simulink library "AVE_Library"  (R2025b)
settings: Solver=VariableStepAuto  StartTime=0.0  StopTime=10.0  RelTol=1e-3
undefined symbols (not defined in the file or in its folder): DiscIntNeverNeededParam
libraries: simulink x44, etargetslib x18, $bdroot x13, GenericTarget x2
(part 2 of 5)

== system AVE_Library/Essential/Transformation ==
  Euler ZYX To Quaternion : Subsystem
      mask help: Convert Euler angles (ZYX-convention) to a unit quaternion. The order of the output quaternion is [W; XYZ], where W denotes the scalar part and XYZ denotes the vector part of the quaternion, respectively. The output quaternion indicates a rotation from b-frame to n-frame.
      mask DialogControl DescGroupVar Prompt: Euler (ZYX) To Quaternion
      mask Display: text(0.5, 0.5, 'Euler (ZYX)\nTo\nQuaternion', 'horizontalAlignment', 'center');
  Euler ZYX To Rotation Matrix : Subsystem
      mask help: Calculate the rotation matrix for a given roll, pitch and yaw angle (ZYX convention).
      mask DialogControl DescGroupVar Prompt: EulerZYXToRotationMatrix
      mask Display: disp('Euler (ZYX)\nTo\nRotation Matrix');
  LLA To NED : Subsystem
      mask help:
      | Convert LLA coordinates (WGS84) to local NED frame coordinates. This implementation uses the algorithm proposed by<br>
      | <i>S. P. Drake,
      | Converting GPS Coordinates to Navigation Coordinates,
      | Surveillance Systems Division, Electronics and Surveillance Research Laboratory, DSTO-TN-0432
      | April, 2002</i><br><br>
      |
      | <b>lat</b><br>Latitude (rad) of position that should be converted to NED.<br><br>
      | <b>lon</b><br>Longitude (rad) of position that should be converted to NED.<br><br>
      | <b>alt</b><br>Altitude (m, positive upwards) of position that should be converted to NED.<br><br>
      | <b>originLat</b><br>Latitude (rad) that indicates the origin of the local NED frame.<br><br>
      | <b>originLon</b><br>Longitude (rad) that indicates the origin of the local NED frame.<br><br>
      | <b>originAlt</b><br>Altitude (m, positive upwards) that indicates the origin of the local NED frame.
      mask DialogControl DescGroupVar Prompt: LLA To NED
      mask Display:
      | % Get dimension of block
      | pos = get_param(gcb, 'Position');
      | width = pos(3) - pos(1);
      | height = pos(4) - pos(2);
      | 
      | % Set image to center of block
      | image('AVE_Icon_LLA2NED.svg');
  LLA To NED Vector : Subsystem
      mask help:
      | Convert LLA coordinates (WGS84) to local NED frame coordinates. This implementation uses the algorithm proposed by<br>
      | <i>S. P. Drake,
      | Converting GPS Coordinates to Navigation Coordinates,
      | Surveillance Systems Division, Electronics and Surveillance Research Laboratory, DSTO-TN-0432
      | April, 2002</i><br><br>
      |
      | <b>positionLLA</b><br>Latitude (rad), longitude (rad) and altitude (m, positive upwards) of position that should be converted to NED.<br><br>
      | <b>originLLA</b><br>Latitude (rad), longitude (rad) and altitude (m, positive upwards) that indicates the origin of the local NED frame.
      mask DialogControl DescGroupVar Prompt: LLA To NED Vector
      mask Display:
      | % Get dimension of block
      | pos = get_param(gcb, 'Position');
      | width = pos(3) - pos(1);
      | height = pos(4) - pos(2);
      | 
      | % Set image to center of block
      | image('AVE_Icon_LLA2NEDVector.svg');
  NED To LLA : Subsystem
      mask help:
      | Convert local NED frame coordinates to LLA coordinates (WGS84). The altitude output is positive upwards.<br>
      | <br>
      | <b>N</b><br>North value of the NED position (m).<br><br>
      | <b>E</b><br>East value of the NED position (m).<br><br>
      | <b>D</b><br>Down value of the NED position (m).<br><br>
      | <b>originLat</b><br>Latitude (rad) that indicates the origin of the local NED frame.<br><br>
      | <b>originLon</b><br>Longitude (rad) that indicates the origin of the local NED frame.<br><br>
      | <b>originAlt</b><br>Altitude (m, positive upwards) that indicates the origin of the local NED frame.
      mask DialogControl DescGroupVar Prompt: NED To LLA
      mask Display:
      | % Get dimension of block
      | pos = get_param(gcb, 'Position');
      | width = pos(3) - pos(1);
      | height = pos(4) - pos(2);
      | 
      | % Set image to center of block
      | image('AVE_Icon_NED2LLA.svg');
  NED To LLA Vector : Subsystem
      mask help:
      | Convert local NED frame coordinates to LLA coordinates (WGS84). The altitude output is positive upwards.<br>
      | <br>
      | <b>positionNED</b><br>North, east and down value of the NED position (m).<br><br>
      | <b>originLLA</b><br>Latitude (rad), longitude (rad) and altitude (m, positive upwards) that indicates the origin of the local NED frame.
      mask DialogControl DescGroupVar Prompt: NED To LLA Vector
      mask Display:
      | % Get dimension of block
      | pos = get_param(gcb, 'Position');
      | width = pos(3) - pos(1);
      | height = pos(4) - pos(2);
      | 
      | % Set image to center of block
      | image('AVE_Icon_NED2LLAVector.svg');
  Quaternion To Euler ZYX : Subsystem
      mask help: Convert a unit quaternion to euler angles. The input quaternion indicates a rotation from b-frame to n-frame and is normalized by this function. The convention of rotation used is ZYX. The order of the input quaternion is [W; XYZ], where W denotes the scalar part and XYZ denotes the vector part of the quaternion, respectively.
      mask DialogControl DescGroupVar Prompt: Quaternion To Euler (ZYX)
      mask Display: text(0.5, 0.5, 'Quaternion\nTo\nEuler (ZYX)', 'horizontalAlignment', 'center');
  Quaternion To Rotation Matrix : Subsystem
      mask help: Convert a unit quaternion to a rotation matrix. The input quaternion indicates a rotation from b-frame to n-frame and is normalized by this function. The order of the input quaternion is [W; XYZ], where W denotes the scalar part and XYZ denotes the vector part of the quaternion, respectively. The output matrix indicates the rotation matrix from b-frame to n-frame.
      mask DialogControl DescGroupVar Prompt: Quaternion To Rotation Matrix
      mask Display: disp('Quaternion\nTo\nRotation Matrix');
  Transform Sensor Euler ZYX : Subsystem
      mask help:
      | Transform an orientation measurement given as euler angles (ZYX-convention) from the sensor-frame to the body frame.<br><br>
      | <b>rollSensor</b><br>Roll angle measurement of the sensor in rad w.r.t. the navigation frame, given in the sensor frame.<br><br>
      | <b>pitchSensor</b><br>Pitch angle measurement of the sensor in rad w.r.t. the navigation frame, given in the sensor frame.<br><br>
      | <b>yawSensor</b><br>Yaw angle measurement of the sensor in rad w.r.t. the navigation frame, given in the sensor frame.<br><br>
      | <b>R_b2s</b><br>Rotation matrix representing the rotation from body-frame to sensor-frame.<br><br>
      mask DialogControl DescGroupVar Prompt: Transform Sensor Velocity PQR
      mask Display: disp('Transform\nSensor\nEuler (ZYX)');
  Transform Sensor Position LLA : Subsystem
      mask help:
      | Transform a geographic position (WGS84) from sensor coordinates to a body-frame, e.g. GPS measurement to body origin.<br><br>
      | <b>latSensor</b><br>Latitude measurement of the sensor in radians.<br><br>
      | <b>lonSensor</b><br>Longitude measurement of the sensor in radians.<br><br>
      | <b>altSensor</b><br>Altitude measurement of the sensor in meters (positive upwards).<br><br>
      | <b>R_b2n</b><br>Rotation matrix representing the rotation from body-frame to navigation frame.<br><br>
      | <b>r_b2s</b><br>Vector that indicates the sensor position w.r.t. the body frame in body frame coordinates (meters).<br><br>
      mask DialogControl DescGroupVar Prompt: Transform Sensor Position LLA
      mask Display: disp('Transform\nSensor\nPosition');
  Transform Sensor Quaternion WXYZ : Subsystem
      mask help:
      | Transform a unit quaternion measurement from a sensor-frame to a body-frame.<br><br>
      | <table border="1" align="center" width="100%"><tr><th>Input</th></tr></table><br><br>
      | <b>quaternionSensor</b><br>
      | Input quaternion from sensor, representing orientation from sensor-frame with respect to navigation-frame.<br><br>
      |
      | <b>R_b2s</b><br>
      | 3-by-3 rotation matrix representing the rotation from body-frame to sensor-frame.<br><br>
      |
      | <table border="1" align="center" width="100%"><tr><th>Output</th></tr></table><br><br>
      | <b>quaternionBody</b><br>
      | Output unit quaternion in body-frame, representing the orientation from the body-frame with respect to the navigation frame.<br><br>
      mask DialogControl DescGroupVar Prompt: Transform Sensor Quaternion WXYZ
      mask Display: disp('Transform\nSensor\nQuaternion');
  Transform Sensor Velocity PQR : Subsystem
      mask help:
      | Transform an angular velocity measurement from a sensor-frame to a body-frame.<br><br>
      | <b>pSensor</b><br>P velocity measurement of the sensor in rad/s w.r.t. navigation frame.<br><br>
      | <b>qSensor</b><br>Q velocity measurement of the sensor in rad/s w.r.t. navigation frame.<br><br>
      | <b>rSensor</b><br>R velocity measurement of the sensor in rad/s w.r.t. navigation frame.<br><br>
      | <b>R_b2s</b><br>Rotation matrix representing the rotation from body-frame to sensor-frame.<br><br>
      mask DialogControl DescGroupVar Prompt: Transform Sensor Velocity PQR
      mask Display: disp('Transform\nSensor\nVelocity (PQR)');
  Transform Sensor Velocity UVW : Subsystem
      mask help:
      | Transform a velocity measurement from a sensor-frame to a body-frame, e.g. DVL measurement to body origin.<br><br>
      | <b>uSensor</b><br>U velocity measurement of the sensor in m/s w.r.t. navigation frame.<br><br>
      | <b>vSensor</b><br>V velocity measurement of the sensor in m/s w.r.t. navigation frame.<br><br>
      | <b>wSensor</b><br>W velocity measurement of the sensor in m/s w.r.t. navigation frame.<br><br>
      | <b>r_b2s</b><br>Vector that indicates the sensor position w.r.t. the body frame in body frame coordinates (meters).<br><br>
      | <b>R_b2s</b><br>Rotation matrix representing the rotation from body-frame to sensor-frame.<br><br>
      | <b>pqr</b><br>Vector of angular velocities in rad/s (angular rate of body-frame w.r.t. navigation-frame in b-frame coordinates).<br><br>
      mask DialogControl DescGroupVar Prompt: Transform Sensor Velocity UVW
      mask Display: disp('Transform\nSensor\nVelocity (UVW)');
  Yaw To Rotation Matrix : Subsystem
      mask help: Create 2-by-2 rotation matrix from given yaw angle. The output rotation matrix represents a transformation from body to navigation frame.
      mask DialogControl DescGroupVar Prompt: Yaw To Rotation Matrix
      mask Display: disp('Yaw\nTo\nRotation Matrix (2x2)');

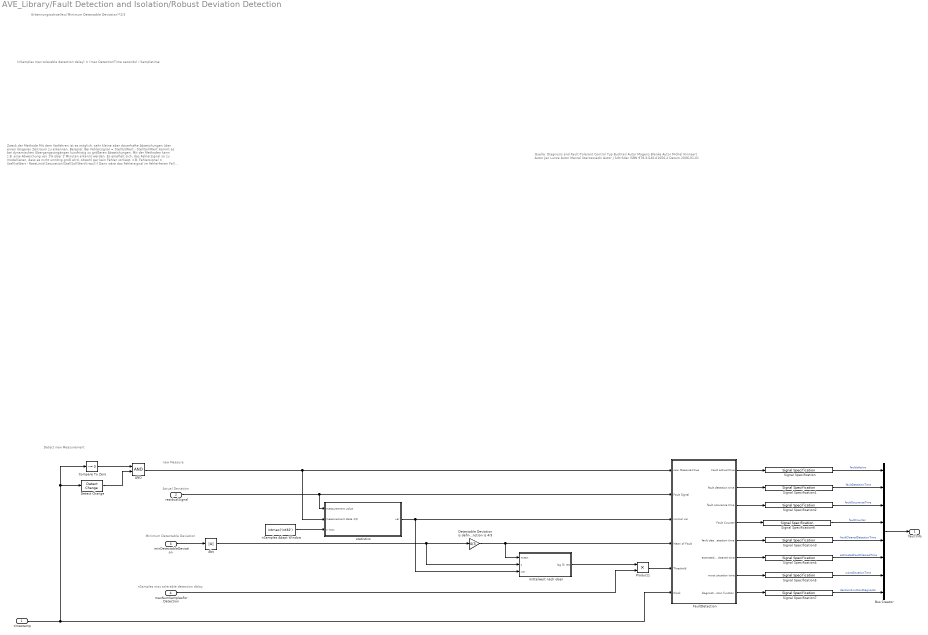
== system AVE_Library/Fault Detection and Isolation/Robust Deviation Detection ==
  note: new Measure
  note: nSamples max tolerable detection delay
  note: Minimum Detectable Deviation
  note: Quelle:
      | Diagnosis and Fault-Tolerant Control
      | Typ Buchteil
      | Autor Mogens Blanke
      | Autor Michel Kinnaert
      | Autor Jan Lunze
      | Autor Marcel Staroswiecki
      | Autor J Schröder
      | ISBN 978-3-540-01056-2
      | Datum 2006-01-01
  note: Zweck der Methode
      | Mit dem Verfahren ist es möglich, sehr kleine aber dauerhafte Abweichungen über einen längeren Zeitraum zu erkennen.
      | Beispiel: Bei
      | Fehlersignal = StellIstWert - StellSollWert
      | kommt es bei dynamischen Übergangsvorgängen kurzfristig zu größeren Abweichungen. Mit der Methoden kann z.B. eine Abweichung von 1% über 2 Minuten erkannt werden.
      | Es empfielt sich, das Fehlersignal so zu modellieren, dass es nicht unnötig groß wird, obwohl gar kein Fehler vorliegt. z.B.
      | Fehlersignal = StellIstWert - RateLimit(Saturation(StellSollWert(t-tau)))
      | Dann wäre das Fehlersignal im fehlerfreien Fall eher nahe null und eine Fehlererkennung zuverlässiger, bzw. sensibler einstellbar.
      |
      | Anleitung für Eingänge
      | Der Eingang "new Measure" soll nur dann auf true gesetzt werden, wenn eine Auswertung des Fehlersignals Sinn ergibt. Das ist zb. dann der Fall, wenn ein neuer Messwert vorliegt. Wenn z.B. ein Antrieb überwacht werden soll, dann nur, wenn der Antrieb tatsächlich läuft. Sonst ist keine Aussage über den (Fehler)Zustand möglich.
      |
      | Das Fehlersignal sollte im fehlerfreien Fall um den Mittelwert 0 schwanken.
      | Im Fehlerfall kommt es zu einer bleibenden möglicherweise kleinen Abweichung nach oben oder unten.
      | Vom Fehlersignal darf nicht der Betrag eingespeist werden! denn das Fehlersignal sollte möglichst normalverteilt sein.
      | "Minimum Detectable Deviation" ist die Abweichung, die sicher detektiert wird.
      | Die Erkennungsschwelle liegt bei 2/3 von diesem Wert.
      | "nSamples max tolerable detection delay" ist die Anzahl an Messwerten, die verarbeitet werden, bis eine Abweichung von "Minimum Detectable Deviation" erkannt wird.
      | Umso größer "nSamples max tolerable detection delay" gewählt wird, desto weniger kommt es zu Fehlererkennungen.
      | Umso größer "Minimum Detectable Deviation" gewählt wird, desto weniger kommt es zu Fehlererkennungen.
      | "Time" dient nur als Grundlage für die ausgegebene Fault detection Time etc.. Man kann die Simulationszeit (clock) nehmen oder eine externe Uhr.
      |
      | Ausgänge
      | "Fault active=true" wenn aktuell ein Fehler aktiv ist.
      | "Fault Counter "Ein neue Fehler wird nur dann hoch gezählt, wenn zwischendurch "Fehlerfreiheit" festgestellt wurde.
      | "worst situation time" gibt den Zeitpunkt an, der bisher am ehesten nach einen Fehlerfall ausgesehen hat.
      |
      | Wenn ein Fehlerhafte Abeichung auftritt dauert es besonders bei kleinen Abweichungen eine Weile, bis dies festgestellt wird. Sobald ein Fehler erkannt wird, geht "Fault active=true" und
      | "fault detection time" wir auf den zuletzt erkannten Fehler aktualisiert.
      | Mit der Methode kann zusätzlich eine Schätzung abgegeben werden, wann der Fehler tatächlich aufgetreten sein könnte. Das ist
      | "fault occurence time" Schätzung eines früheren Zeitpunktes, wann der Fehler wahrscheinlich aufgetreten ist.
      | Wenn der Fehler scheinbar nicht mehr aktiv ist, geht "Fault active=false" und die Werte für
      | "fault cleared detection time" Zeitpunkt, bei dem Normalbeitrieb erkannt wurde
      | "estmated fault cleared time" früherer Zeitpunkt, bei dem Normalbeitrieb wahrscheinlich schon eintetreten ist.
      |
      | Mit dem Diagnostic-Signal
      | "decision function (diagnostic)" kann überprüft werden, wie kurz vor einem Alarm/Fehlalarm die Auswertung liegt.
      | Das gezeigt Signal steigt bei Wahrscheinlichkeit für einen Alarm an und bewegt sich Richtung null, wenn Fehlerfreiheit vorliegt.
      | Sobald der eingezeichnete Threshold überschritten ist, wird eine Fehlererkennung ausgelöst.
  note: Detect new Measurement
  note: Erkennungsschwelle=(Minimum Detectable Deviation)*2/3
  note: (nSamples max tolerable detection delay) = (max DetectionTime seconds) / Sampletime
  note: Actual Deviation
  timestamp : Inport
  residualSignal : Inport  Port=2
  minDetectableDeviation : Inport  Port=3
  maxNumSamplesForDetection : Inport  Port=4
  AND : Logic  AllPortsSameDT=off  OutDataTypeStr=boolean
  Abs : Abs  SaturateOnIntegerOverflow=off
  Bus Creator : BusCreator  Inputs=8
  Compare To Zero : simulink/Logic and Bit Operations/Compare To Zero  relop=~=  OutDataTypeStr=boolean
  Detect Change : simulink/Logic and Bit Operations/Detect Change  vinit=0  OutDataTypeStr=boolean
  Detectable Deviation is defined to locate between intersection and mean of fault propability density function is 4/3 : Gain  Gain=4/3
  FaultDetection : Subsystem
  Product1 : Product
  Signal Specification : SignalSpecification  OutDataTypeStr=boolean
  Signal Specification{1..5} (5 alike) : SignalSpecification  OutDataTypeStr=double  Unit=s
  Signal Specification6 : SignalSpecification  OutDataTypeStr=uint32
  Signal Specification7 : SignalSpecification  OutDataTypeStr=double
  mittelwert nach oben : Subsystem
  nSamples Adapt Window : Constant  Value=intmax('int32')
  statistics : Subsystem
  faultInfo : Outport
  wires:
  Bus Creator/1 -> faultInfo/1
  Signal Specification7/1 -> Bus Creator/8  "decisionFunctionDiagnostic"
  Signal Specification6/1 -> Bus Creator/4  "faultCounter"
  Signal Specification5/1 -> Bus Creator/7  "worstSituationTime"
  Signal Specification4/1 -> Bus Creator/6  "estimatedFaultClearedTime"
  Signal Specification3/1 -> Bus Creator/5  "faultClearedDetectionTime"
  Signal Specification2/1 -> Bus Creator/3  "faultOccurenceTime"
  Signal Specification1/1 -> Bus Creator/2  "faultDetectionTime"
  Signal Specification/1 -> Bus Creator/1  "faultIsActive"
  Compare To Zero/1 -> AND/1
  timestamp/1 -> Detect Change/1, Compare To Zero/1, FaultDetection/6(Clock)
  Detect Change/1 -> AND/2
  FaultDetection/7(worst situation time) -> Signal Specification5/1
  FaultDetection/5(fault cleared detection time) -> Signal Specification3/1
  FaultDetection/6(estmated fault cleared time) -> Signal Specification4/1
  Abs/1 -> mittelwert nach oben/2(z), Detectable Deviation is defined to locate between intersection and mean of fault propability density function is 4/3/1
  Detectable Deviation is defined to locate between intersection and mean of fault propability density function is 4/3/1 -> mittelwert nach oben/1(mean), FaultDetection/4(Mean of Fault)
  FaultDetection/2(fault detection time) -> Signal Specification1/1
  mittelwert nach oben/1(log lik rat) -> Product1/1
  nSamples Adapt Window/1 -> statistics/3(n max)
  Product1/1 -> FaultDetection/5(Threshold)
  maxNumSamplesForDetection/1 -> Product1/2
  statistics/1(var) -> mittelwert nach oben/3(var), FaultDetection/3(normal var)
  minDetectableDeviation/1 -> Abs/1
  residualSignal/1 -> statistics/1(measurement value), FaultDetection/2(Fault Signal)
  FaultDetection/4(Fault Counter) -> Signal Specification6/1
  AND/1 -> statistics/2(measurement state 1/0), FaultDetection/1(new Measure=true)
  FaultDetection/8(diagnostic decision function) -> Signal Specification7/1
  FaultDetection/1(Fault active=true) -> Signal Specification/1
  FaultDetection/3(fault occurence time) -> Signal Specification2/1

== system AVE_Library/Guidance/Trajectory Track Error ==
  time : Inport  OutDataTypeStr=double  Unit=s  PortDimensions=1
  positionLLA : Inport  Port=2  OutDataTypeStr=double  PortDimensions=3
  matTimeLatLon : Inport  Port=3  OutDataTypeStr=double
  numPoints : Inport  Port=4  PortDimensions=1
  Data Type Conversion : DataTypeConversion  OutDataTypeStr=int32  SaturateOnIntegerOverflow=off  RndMeth=Floor
  Data Type Conversion1 : DataTypeConversion  OutDataTypeStr=int32  SaturateOnIntegerOverflow=off  RndMeth=Floor
  Data Type Conversion2 : DataTypeConversion  OutDataTypeStr=int32  SaturateOnIntegerOverflow=off  RndMeth=Floor
  Data Type Conversion3 : DataTypeConversion  OutDataTypeStr=boolean  SaturateOnIntegerOverflow=off  RndMeth=Floor
  MATLAB Function1 : MATLAB Function  TreatAsAtomicUnit=on
  valid : Outport  OutDataTypeStr=boolean  PortDimensions=1
  trackError : Outport  Port=2  OutDataTypeStr=double  Unit=m  PortDimensions=2
  closestSegmentIndices : Outport  Port=3  OutDataTypeStr=int32  PortDimensions=2
  closestSegmentLinearInterpolationRatio : Outport  Port=4  OutDataTypeStr=double  PortDimensions=1
  targetSegmentIndices : Outport  Port=5  OutDataTypeStr=int32  PortDimensions=2
  targetSegmentLinearInterpolationRatio : Outport  Port=6  OutDataTypeStr=double  PortDimensions=1
  wires:
  MATLAB Function1/6(targetSegmentLinearInterpolationRatio) -> targetSegmentLinearInterpolationRatio/1
  MATLAB Function1/5(targetSegmentIndices) -> Data Type Conversion2/1
  MATLAB Function1/3(closestSegmentIndices) -> Data Type Conversion1/1
  MATLAB Function1/2(trackError) -> trackError/1
  matTimeLatLon/1 -> MATLAB Function1/3(matTimeLatLon)
  numPoints/1 -> Data Type Conversion/1
  MATLAB Function1/4(closestSegmentLinearInterpolationRatio) -> closestSegmentLinearInterpolationRatio/1
  positionLLA/1 -> MATLAB Function1/2(positionLLA)
  time/1 -> MATLAB Function1/1(time)
  MATLAB Function1/1(valid) -> Data Type Conversion3/1
  Data Type Conversion/1 -> MATLAB Function1/4(numPoints)
  Data Type Conversion1/1 -> closestSegmentIndices/1
  Data Type Conversion2/1 -> targetSegmentIndices/1
  Data Type Conversion3/1 -> valid/1

== system AVE_Library/Navigation/Sensor Preprocessing ==
  Butterworth Filter : Subsystem  mask{numZeros=0, numPoles=1}
      mask prompts: numZeros "Number of derivations:"; numPoles "Order of low pass:"
      mask help:
      | A butterworth filter where the timeconstant can be changed online using the input <b>T</b>. If this input is changed, the internal filter is to be reset.
      | The order of the filter (order of low pass and number of derivations) is set by the mask parameters.
      mask DialogControl DescGroupVar Prompt: Butterworth Filter
      mask Display: disp('Butterworth Filter')
  Detect Outliers 1D : Subsystem
      mask help: Detect an outlier based on the previous data value. If the absolute difference of the data to the previous valid data is greater than a given threshold, then the number of outliers is incremented. The number of outliers is reset to zero if either the data is in the valid range again or the number of outliers exceeds the specified maximum number of outliers.
      mask DialogControl DescGroupVar Prompt: Detect Outliers 1D
      mask Display: disp('Detect Outliers\n1D');
  Detect Outliers Angle 1D : Subsystem
      mask help: Detect an outlier based on the previous data value. If the absolute difference of the data to the previous valid data is greater than a given threshold, then the number of outliers is incremented. The number of outliers is reset to zero if either the data is in the valid range again or the number of outliers exceeds the specified maximum number of outliers.
      mask DialogControl DescGroupVar Prompt: Detect Outliers Angle 1D
      mask Display: disp('Detect Outliers\nAngle 1D');
  Detect Outliers GNSS : Subsystem
      mask help: Detect a GNSS outlier based on the previous position data. If the absolute difference of the position to the previous valid position is greater than a given threshold, then the number of outliers is incremented. The number of outliers is reset to zero if either the position is in the valid range again or the number of outliers exceeds the specified maximum number of outliers. The threshold is separated into a horizontal threshold and a vertical threshold.
      mask DialogControl DescGroupVar Prompt: Detect Outliers GNSS
      mask Display: disp('Detect Outliers\nGNSS');
  Smoothed Quaternion Time Derivative : Subsystem
      mask help: The time derivate of the input quaternion is calculated to compute the angular velocity. The input quaternion must indicate a rotation from body-frame to navigation frame. The elements are [qw; qx; qy; qz] where qw denotes the scalar part and [qx; qy; qz] denotes the vector part of the unit quaternion. The input quaternion is filtered by a first order low pass that only calculates new output values if the trigger input is high. The time input is used to calculate the elapsed time to a previous trigger event. Internally, the trapezoidal rule is used as integration method for the discrete filter design. The filtered input quaternion is then used to calculate the time derivate.
      mask DialogControl DescGroupVar Prompt: Smoothed Quaternion Time Derivative
      mask Display: disp('Smoothed Quaternion Time Derivative\nto\nAngular Velocity');
  Triggered Low Pass : Subsystem
      mask help: A first order low pass filter that only calculates new output values if the trigger input is high. The time input is used to calculate the elapsed time to a previous trigger event. Internally, the trapezoidal rule is used as integration method for the discrete filter design.
      mask DialogControl DescGroupVar Prompt: Triggered Low Pass
      mask Display: disp('Triggered\nLow Pass');

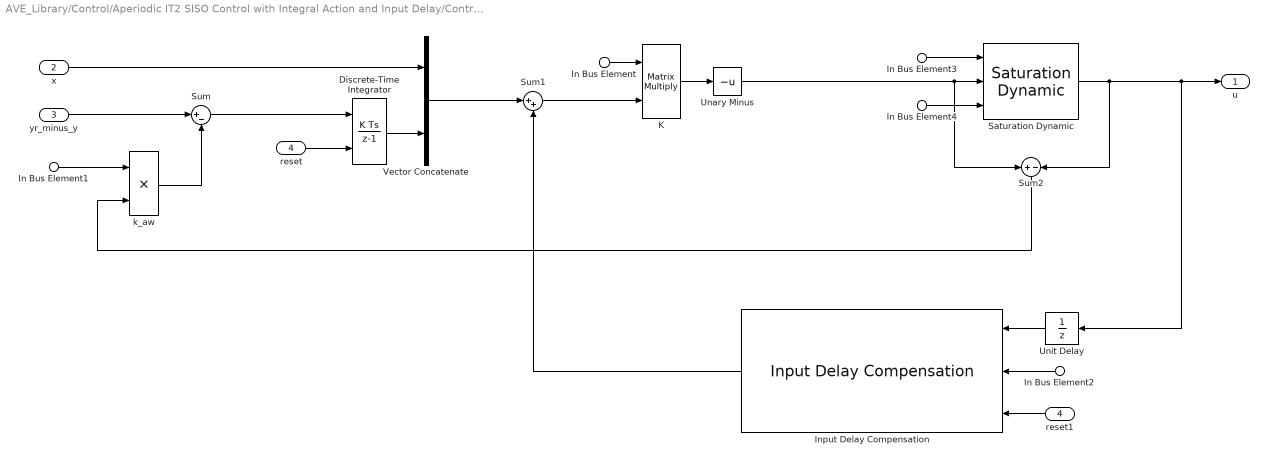
== system AVE_Library/Control/Aperiodic IT2 SISO Control with Integral Action and Input Delay/Controller ==
  In Bus Element : Inport  PortName=controllerDesign  Element=K
  In Bus Element1 : Inport  PortName=controllerDesign  Element=antiWindupGain
  In Bus Element2 : Inport  PortName=controllerDesign  Element=delayWeights
  In Bus Element3 : Inport  PortName=controllerDesign  Element=upperLimit
  In Bus Element4 : Inport  PortName=controllerDesign  Element=lowerLimit
  x : Inport  Port=2
  yr_minus_y : Inport  Port=3
  reset : Inport  Port=4
  Discrete-Time Integrator : DiscreteIntegrator  ExternalReset=level  SampleTime=SampleTime  ICPrevOutput=DiscIntNeverNeededParam  ICPrevScaledInput=DiscIntNeverNeededParam
  Input Delay Compensation : $bdroot/Control/Input Delay Compensation  dimU=1  dimX=4  maxNumDelays=maxNumDelays  SampleTime=SampleTime
  K : Product  Multiplication=Matrix(*)
  Saturation Dynamic : simulink/Discontinuities/Saturation Dynamic  OutMin=[]  OutMax=[]  OutDataTypeStr=Inherit: Same as second input  OutDataType=fixdt(1, 16)  OutScaling=2^-10  DoSatur=off
  Sum : Sum  Inputs=|+-
  Sum1 : Sum  Inputs=|++
  Sum2 : Sum  Inputs=+-
  Unary Minus : UnaryMinus
  Unit Delay : UnitDelay  SampleTime=SampleTime  HasFrameUpgradeWarning=on
  Vector Concatenate : Concatenate
  k_aw : Product
  reset1 : InportShadow  Port=4
  u : Outport
  wires:
  In Bus Element4/1 -> Saturation Dynamic/3
  In Bus Element3/1 -> Saturation Dynamic/1
  Sum2/1 -> k_aw/2
  Unit Delay/1 -> Input Delay Compensation/1
  Saturation Dynamic/1 -> u/1, Unit Delay/1, Sum2/2
  reset1/1 -> Input Delay Compensation/3
  In Bus Element2/1 -> Input Delay Compensation/2
  Input Delay Compensation/1 -> Sum1/2
  In Bus Element1/1 -> k_aw/1
  Sum1/1 -> K/2
  In Bus Element/1 -> K/1
  reset/1 -> Discrete-Time Integrator/2
  Unary Minus/1 -> Saturation Dynamic/2, Sum2/1
  Discrete-Time Integrator/1 -> Vector Concatenate/2
  yr_minus_y/1 -> Sum/1
  Sum/1 -> Discrete-Time Integrator/1
  k_aw/1 -> Sum/2
  Vector Concatenate/1 -> Sum1/1
  x/1 -> Vector Concatenate/1
  K/1 -> Unary Minus/1

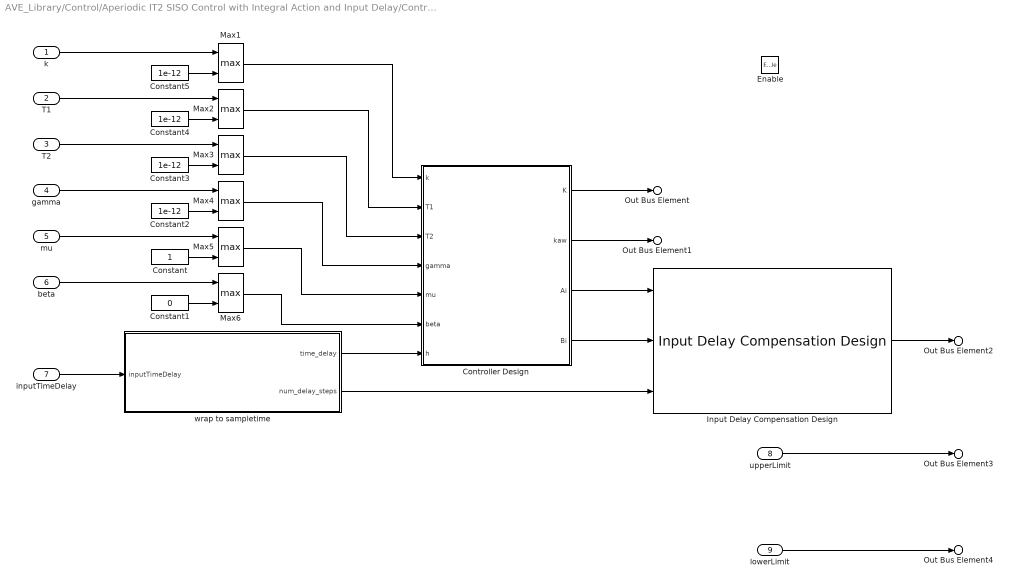
== system AVE_Library/Control/Aperiodic IT2 SISO Control with Integral Action and Input Delay/Controller Design ==
  k : Inport
  T1 : Inport  Port=2
  T2 : Inport  Port=3
  gamma : Inport  Port=4
  mu : Inport  Port=5
  beta : Inport  Port=6
  inputTimeDelay : Inport  Port=7
  upperLimit : Inport  Port=8
  lowerLimit : Inport  Port=9
  Enable : EnablePort
  Constant : Constant
  Constant1 : Constant  Value=0
  Constant{2..5} (4 alike) : Constant  Value=1e-12
  Controller Design : MATLAB Function  TreatAsAtomicUnit=on
  Input Delay Compensation Design : $bdroot/Control/Input Delay Compensation Design  dimU=1  dimX=4  maxNumDelays=maxNumDelays  SampleTime=SampleTime
  Max{1..6} (6 alike) : MinMax  Function=max  Inputs=2
  wrap to sampletime : MATLAB Function  TreatAsAtomicUnit=on
  Out Bus Element : Outport  PortName=controllerDesign  Element=K
  Out Bus Element1 : Outport  PortName=controllerDesign  Element=antiWindupGain
  Out Bus Element2 : Outport  PortName=controllerDesign  Element=delayWeights
  Out Bus Element3 : Outport  PortName=controllerDesign  Element=upperLimit
  Out Bus Element4 : Outport  PortName=controllerDesign  Element=lowerLimit
  wires:
  Max1/1 -> Controller Design/1(k)
  Max2/1 -> Controller Design/2(T1)
  Max3/1 -> Controller Design/3(T2)
  Max4/1 -> Controller Design/4(gamma)
  Max5/1 -> Controller Design/5(mu)
  Max6/1 -> Controller Design/6(beta)
  beta/1 -> Max6/1
  mu/1 -> Max5/1
  gamma/1 -> Max4/1
  T2/1 -> Max3/1
  T1/1 -> Max2/1
  k/1 -> Max1/1
  Constant5/1 -> Max1/2
  Constant4/1 -> Max2/2
  Constant3/1 -> Max3/2
  Constant2/1 -> Max4/2
  Constant1/1 -> Max6/2
  Constant/1 -> Max5/2
  inputTimeDelay/1 -> wrap to sampletime/1(inputTimeDelay)
  Controller Design/2(kaw) -> Out Bus Element1/1
  Controller Design/1(K) -> Out Bus Element/1
  wrap to sampletime/1(time_delay) -> Controller Design/7(h)
  Controller Design/4(Bi) -> Input Delay Compensation Design/2
  wrap to sampletime/2(num_delay_steps) -> Input Delay Compensation Design/3
  Input Delay Compensation Design/1 -> Out Bus Element2/1
  Controller Design/3(Ai) -> Input Delay Compensation Design/1
  upperLimit/1 -> Out Bus Element3/1
  lowerLimit/1 -> Out Bus Element4/1

== system AVE_Library/Control/Aperiodic IT2 SISO Control with Integral Action and Input Delay/set limits ==
  saturationLimits : Inport
  Demux : Demux  Outputs=2
  Max : MinMax  Function=max  Inputs=2
  Min : MinMax  Inputs=2
  upperLimit : Outport
  lowerLimit : Outport  Port=2
  wires:
  Demux/1 -> Min/1, Max/1
  Demux/2 -> Max/2, Min/2
  Min/1 -> lowerLimit/1
  Max/1 -> upperLimit/1
  saturationLimits/1 -> Demux/1

== system AVE_Library/Essential/Check For Timeout UTC/Enabled Subsystem ==
  In1 : Inport
  Enable : EnablePort
  Out1 : Outport  InitialOutput=-2*timeout
  wires:
  In1/1 -> Out1/1

== system AVE_Library/Essential/Equations of Motion/Kinematic 3DoF Euclidean ==
  uvr : Inport  OutDataTypeStr=double  PortDimensions=3
  initialPoseXYPsi : Inport  Port=2  OutDataTypeStr=double  PortDimensions=3
  reset : Inport  Port=3  OutDataTypeStr=boolean  PortDimensions=1
  Demux : Demux  Outputs=3
  Integrator : Integrator  ExternalReset=level  InitialConditionSource=external
  Mux : Mux  Inputs=3
  Product : Product  Multiplication=Matrix(*)
  Selector : Selector  InputPortWidth=3  IndexOptions=Index vector (dialog)  Indices=1:2  OutputSizes=1
  Selector1 : Selector  InputPortWidth=3  IndexOptions=Index vector (dialog)  Indices=3  OutputSizes=1
  Selector2 : Selector  InputPortWidth=3  IndexOptions=Index vector (dialog)  Indices=3  OutputSizes=1
  Symmetrical Angle : $bdroot/Essential/Symmetrical Angle
  Vector Concatenate : Concatenate
  Yaw To Rotation Matrix : $bdroot/Essential/Transformation/Yaw To Rotation Matrix
      settings: LibrarySourceBlock=AVControl/Transformation/Yaw To Rotation Matrix
  poseXYPsi : Outport  OutDataTypeStr=double  PortDimensions=3
  wires:
  reset/1 -> Integrator/2
  initialPoseXYPsi/1 -> Integrator/3
  Vector Concatenate/1 -> Integrator/1
  Product/1 -> Vector Concatenate/1
  Selector/1 -> Product/2
  Selector1/1 -> Vector Concatenate/2
  uvr/1 -> Selector1/1, Selector/1
  Yaw To Rotation Matrix/1 -> Product/1
  Integrator/1 -> Demux/1
  Demux/3 -> Symmetrical Angle/1
  Demux/1 -> Mux/1
  Demux/2 -> Mux/2
  Symmetrical Angle/1 -> Mux/3
  Mux/1 -> Selector2/1, poseXYPsi/1
  Selector2/1 -> Yaw To Rotation Matrix/1

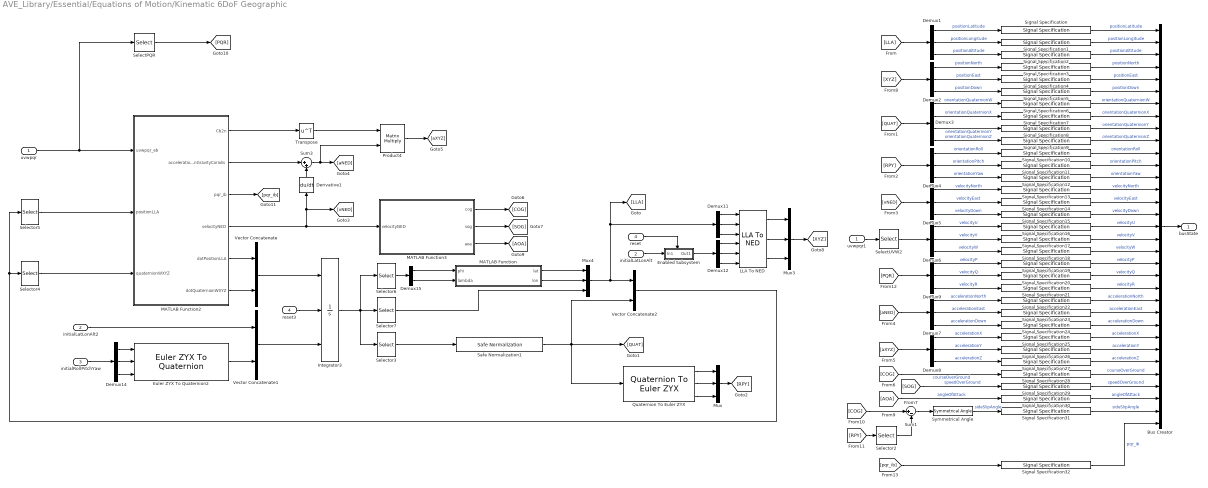
== system AVE_Library/Essential/Equations of Motion/Kinematic 6DoF Geographic ==
  uvwpqr : Inport  OutDataTypeStr=double  PortDimensions=6
  initialLatLonAlt : Inport  Port=2  OutDataTypeStr=double  PortDimensions=3
  initialRollPitchYaw : Inport  Port=3  OutDataTypeStr=double  Unit=rad  PortDimensions=3
  reset : Inport  Port=4  OutDataTypeStr=boolean  PortDimensions=1
  Bus Creator : BusCreator  Inputs=33
  Demux{1..2,4..9,11..12,14} (11 alike) : Demux  Outputs=3
  Demux15 : Demux  Outputs=2
  Demux3 : Demux
  Derivative1 : Derivative
  Enabled Subsystem : Subsystem  TreatAsAtomicUnit=on
  Euler ZYX To Quaternion2 : $bdroot/Essential/Transformation/Euler ZYX To Quaternion
      settings: LibrarySourceBlock=AVControl/Transformation/Euler ZYX To Quaternion
  Integrator3 : Integrator  ExternalReset=level  InitialConditionSource=external
  LLA To NED : $bdroot/Essential/Transformation/LLA To NED
      settings: LibrarySourceBlock=AVControl/Transformation/LLA To NED
  MATLAB Function : MATLAB Function  TreatAsAtomicUnit=on
  MATLAB Function2 : MATLAB Function  TreatAsAtomicUnit=on
  MATLAB Function3 : MATLAB Function  TreatAsAtomicUnit=on
  Mux : Mux  Inputs=3
  Mux3 : Mux  Inputs=3
  Mux4 : Mux  Inputs=3
  Product4 : Product  Multiplication=Matrix(*)
  Quaternion To Euler ZYX : $bdroot/Essential/Transformation/Quaternion To Euler ZYX
      settings: LibrarySourceBlock=AVControl/Transformation/Quaternion To Euler ZYX
  Safe Normalization1 : $bdroot/Essential/Safe Normalization
  SelectPQR : Selector  InputPortWidth=6  IndexOptions=Index vector (dialog)  Indices=[4:6]  OutputSizes=1
  SelectUVW2 : Selector  InputPortWidth=6  IndexOptions=Index vector (dialog)  Indices=[1:3]  OutputSizes=1
  Selector2 : Selector  InputPortWidth=3  IndexOptions=Index vector (dialog)  Indices=3  OutputSizes=1
  Selector3 : Selector  InputPortWidth=7  IndexOptions=Index vector (dialog)  Indices=[4:7]  OutputSizes=1
  Selector4 : Selector  InputPortWidth=7  IndexOptions=Index vector (dialog)  Indices=[4:7]  OutputSizes=1
  Selector5 : Selector  InputPortWidth=7  IndexOptions=Index vector (dialog)  Indices=[1:3]  OutputSizes=1
  Selector6 : Selector  InputPortWidth=7  IndexOptions=Index vector (dialog)  Indices=[1:2]  OutputSizes=1
  Selector7 : Selector  InputPortWidth=7  IndexOptions=Index vector (dialog)  Indices=3  OutputSizes=1
  Signal Specification{,1,10..12,28,30..31} (8 alike) : SignalSpecification  OutDataTypeStr=double  Unit=rad  Dimensions=1
  Signal Specification{13..18,29} (7 alike) : SignalSpecification  OutDataTypeStr=double  Unit=m/s  Dimensions=1
  Signal Specification19 : SignalSpecification  OutDataTypeStr=double  Unit=rad/s  Dimensions=1
  Signal Specification{2..5} (4 alike) : SignalSpecification  OutDataTypeStr=double  Unit=m  Dimensions=1
  Signal Specification20 : SignalSpecification  OutDataTypeStr=double  Unit=rad/s  Dimensions=1
  Signal Specification21 : SignalSpecification  OutDataTypeStr=double  Unit=rad/s  Dimensions=1
  Signal Specification{22..27} (6 alike) : SignalSpecification  OutDataTypeStr=double  Unit=m/s^2  Dimensions=1
  Signal Specification32 : SignalSpecification  OutDataTypeStr=double  Unit=rad/s  Dimensions=3
  Signal Specification{6..9} (4 alike) : SignalSpecification  OutDataTypeStr=double  Dimensions=1
  Sum1 : Sum  Inputs=|+-
  Sum3 : Sum  Inputs=|++
  Symmetrical Angle : $bdroot/Essential/Symmetrical Angle
  Transpose : Math  Operator=transpose
  Vector Concatenate : Concatenate
  Vector Concatenate1 : Concatenate
  Vector Concatenate2 : Concatenate
  initialLatLonAlt2 : InportShadow  Port=2  OutDataTypeStr=double  PortDimensions=3
  reset3 : InportShadow  Port=4  OutDataTypeStr=boolean  PortDimensions=1
  uvwpqr1 : InportShadow  OutDataTypeStr=double  PortDimensions=6
  busState : Outport  VectorParamsAs1DForOutWhenUnconnected=off
  wires:
  Product4/1 -> [aXYZ]
  Transpose/1 -> Product4/1
  Sum3/1 -> [aNED], Product4/2
  Derivative1/1 -> Sum3/2
  [AOA] -> Signal Specification30/1  "angleOfAttack"
  Demux11/3 -> LLA To NED/3
  [aXYZ] -> Demux8/1
  Demux1/1 -> Signal Specification/1  "positionLatitude"
  Demux5/2 -> Signal Specification14/1  "velocityEast"
  Demux2/3 -> Signal Specification5/1  "positionDown"
  Demux5/1 -> Signal Specification13/1  "velocityNorth"
  [vNED] -> Demux5/1
  Demux2/1 -> Signal Specification3/1  "positionNorth"
  Demux6/1 -> Signal Specification16/1  "velocityU"
  LLA To NED/3 -> Mux3/3
  Demux2/2 -> Signal Specification4/1  "positionEast"
  Demux4/3 -> Signal Specification12/1  "orientationYaw"
  Demux3/4 -> Signal Specification9/1  "orientationQuaternionZ"
  Demux7/2 -> Signal Specification23/1  "accelerationEast"
  Mux/1 -> [RPY]
  [RPY] -> Demux4/1
  LLA To NED/2 -> Mux3/2
  Demux6/3 -> Signal Specification18/1  "velocityW"
  Demux8/1 -> Signal Specification25/1  "accelerationX"
  Mux3/1 -> [XYZ]
  Demux12/1 -> LLA To NED/4
  Enabled Subsystem/1(Out1) -> Demux12/1
  Demux6/2 -> Signal Specification17/1  "velocityV"
  [PQR] -> Demux9/1
  Demux4/2 -> Signal Specification11/1  "orientationPitch"
  Demux12/3 -> LLA To NED/6
  [COG] -> Sum1/1
  Demux8/3 -> Signal Specification27/1  "accelerationZ"
  initialLatLonAlt/1 -> Enabled Subsystem/1(In1)
  Demux11/2 -> LLA To NED/2
  Demux3/1 -> Signal Specification6/1  "orientationQuaternionW"
  LLA To NED/1 -> Mux3/1
  Sum1/1 -> Symmetrical Angle/1
  [QUAT] -> Demux3/1
  Demux3/3 -> Signal Specification8/1  "orientationQuaternionY"
  Selector2/1 -> Sum1/2
  [RPY] -> Selector2/1
  Demux7/3 -> Signal Specification24/1  "accelerationDown"
  [COG] -> Signal Specification28/1  "courseOverGround"
  reset/1 -> Enabled Subsystem/Enable
  Bus Creator/1 -> busState/1
  [SOG] -> Signal Specification29/1  "speedOverGround"
  Demux9/1 -> Signal Specification19/1  "velocityP"
  Demux4/1 -> Signal Specification10/1  "orientationRoll"
  [XYZ] -> Demux2/1
  [LLA] -> Demux1/1
  Demux9/3 -> Signal Specification21/1  "velocityR"
  Demux9/2 -> Signal Specification20/1  "velocityQ"
  [aNED] -> Demux7/1
  Demux12/2 -> LLA To NED/5
  Demux11/1 -> LLA To NED/1
  Demux8/2 -> Signal Specification26/1  "accelerationY"
  uvwpqr1/1 -> SelectUVW2/1
  Demux1/3 -> Signal Specification2/1  "positionAltitude"
  SelectUVW2/1 -> Demux6/1
  Demux7/1 -> Signal Specification22/1  "accelerationNorth"
  Quaternion To Euler ZYX/2 -> Mux/2
  Demux3/2 -> Signal Specification7/1  "orientationQuaternionX"
  Demux5/3 -> Signal Specification15/1  "velocityDown"
  Quaternion To Euler ZYX/1 -> Mux/1
  Quaternion To Euler ZYX/3 -> Mux/3
  Demux1/2 -> Signal Specification1/1  "positionLongitude"
  Symmetrical Angle/1 -> Signal Specification31/1  "sideSlipAngle"
  MATLAB Function2/5(dotPositionLLA) -> Vector Concatenate/1
  MATLAB Function2/6(dotQuaternionWXYZ) -> Vector Concatenate/2
  Vector Concatenate/1 -> Integrator3/1
  Demux14/3 -> Euler ZYX To Quaternion2/3
  Demux14/2 -> Euler ZYX To Quaternion2/2
  Demux14/1 -> Euler ZYX To Quaternion2/1
  initialRollPitchYaw/1 -> Demux14/1
  Euler ZYX To Quaternion2/1 -> Vector Concatenate1/2
  initialLatLonAlt2/1 -> Vector Concatenate1/1
  Integrator3/1 -> Selector6/1, Selector3/1, Selector7/1
  Selector3/1 -> Safe Normalization1/1
  Selector4/1 -> MATLAB Function2/3(quaternionWXYZ)
  Selector5/1 -> MATLAB Function2/2(positionLLA)
  Vector Concatenate2/1 -> Selector5/1, Selector4/1
  Vector Concatenate1/1 -> Integrator3/3
  reset3/1 -> Integrator3/2
  uvwpqr/1 -> SelectPQR/1, MATLAB Function2/1(uvwpqr_eb)
  Safe Normalization1/1 -> Vector Concatenate2/2, Quaternion To Euler ZYX/1, [QUAT]
  Demux15/1 -> MATLAB Function/1(phi)
  Demux15/2 -> MATLAB Function/2(lambda)
  Selector6/1 -> Demux15/1
  MATLAB Function3/1(cog) -> [COG]
  MATLAB Function3/2(sog) -> [SOG]
  MATLAB Function3/3(aoa) -> [AOA]
  MATLAB Function2/4(velocityNED) -> Derivative1/1, [vNED], MATLAB Function3/1(velocityNED)
  MATLAB Function/1(lat) -> Mux4/1
  MATLAB Function/2(lon) -> Mux4/2
  Selector7/1 -> Mux4/3
  Mux4/1 -> [LLA], Demux11/1, Vector Concatenate2/1
  MATLAB Function2/2(accelerationGravityCoriolis) -> Sum3/1
  MATLAB Function2/1(Cb2n) -> Transpose/1
  Signal Specification/1 -> Bus Creator/1  "positionLatitude"
  Signal Specification1/1 -> Bus Creator/2  "positionLongitude"
  Signal Specification2/1 -> Bus Creator/3  "positionAltitude"
  Signal Specification3/1 -> Bus Creator/4  "positionNorth"
  Signal Specification4/1 -> Bus Creator/5  "positionEast"
  Signal Specification5/1 -> Bus Creator/6  "positionDown"
  Signal Specification6/1 -> Bus Creator/7  "orientationQuaternionW"
  Signal Specification7/1 -> Bus Creator/8  "orientationQuaternionX"
  Signal Specification8/1 -> Bus Creator/9  "orientationQuaternionY"
  Signal Specification9/1 -> Bus Creator/10  "orientationQuaternionZ"
  Signal Specification10/1 -> Bus Creator/11  "orientationRoll"
  Signal Specification11/1 -> Bus Creator/12  "orientationPitch"
  Signal Specification12/1 -> Bus Creator/13  "orientationYaw"
  Signal Specification13/1 -> Bus Creator/14  "velocityNorth"
  Signal Specification14/1 -> Bus Creator/15  "velocityEast"
  Signal Specification15/1 -> Bus Creator/16  "velocityDown"
  Signal Specification16/1 -> Bus Creator/17  "velocityU"
  Signal Specification17/1 -> Bus Creator/18  "velocityV"
  Signal Specification18/1 -> Bus Creator/19  "velocityW"
  Signal Specification19/1 -> Bus Creator/20  "velocityP"
  Signal Specification20/1 -> Bus Creator/21  "velocityQ"
  Signal Specification21/1 -> Bus Creator/22  "velocityR"
  Signal Specification22/1 -> Bus Creator/23  "accelerationNorth"
  Signal Specification23/1 -> Bus Creator/24  "accelerationEast"
  Signal Specification24/1 -> Bus Creator/25  "accelerationDown"
  Signal Specification25/1 -> Bus Creator/26  "accelerationX"
  Signal Specification26/1 -> Bus Creator/27  "accelerationY"
  Signal Specification27/1 -> Bus Creator/28  "accelerationZ"
  Signal Specification28/1 -> Bus Creator/29  "courseOverGround"
  Signal Specification29/1 -> Bus Creator/30  "speedOverGround"
  Signal Specification30/1 -> Bus Creator/31  "angleOfAttack"
  Signal Specification31/1 -> Bus Creator/32  "sideSlipAngle"
  SelectPQR/1 -> [PQR]
  MATLAB Function2/3(pqr_ib) -> [pqr_ib]
  [pqr_ib] -> Signal Specification32/1
  Signal Specification32/1 -> Bus Creator/33  "pqr_ib"

== system AVE_Library/Essential/Equations of Motion/Strapdown Algorithm ==
  sampletime : Inport  OutDataTypeStr=double  Unit=s  PortDimensions=1
  imuAcceleration : Inport  Port=2  OutDataTypeStr=double  Unit=m/s^2  PortDimensions=3
  imuAngularRate : Inport  Port=3  OutDataTypeStr=double  Unit=rad/s  PortDimensions=3
  positionLLA : Inport  Port=4  OutDataTypeStr=double  PortDimensions=3
  orientationQuaternionWXYZ : Inport  Port=5  OutDataTypeStr=double  PortDimensions=4
  velocityUVW : Inport  Port=6  OutDataTypeStr=double  Unit=m/s  PortDimensions=3
  MATLAB Function : MATLAB Function  TreatAsAtomicUnit=on
  outPositionLLA : Outport  OutDataTypeStr=double  PortDimensions=3
  outOrientationQuaternionWXYZ : Outport  Port=2  OutDataTypeStr=double  PortDimensions=4
  outVelocityUVW : Outport  Port=3  OutDataTypeStr=double  Unit=m/s  PortDimensions=3
  wires:
  positionLLA/1 -> MATLAB Function/4(positionLLA)
  orientationQuaternionWXYZ/1 -> MATLAB Function/5(orientationQuaternionWXYZ)
  velocityUVW/1 -> MATLAB Function/6(velocityUVW)
  MATLAB Function/2(outOrientationQuaternionWXYZ) -> outOrientationQuaternionWXYZ/1
  imuAcceleration/1 -> MATLAB Function/2(imuAcceleration)
  imuAngularRate/1 -> MATLAB Function/3(imuAngularRate)
  MATLAB Function/3(outVelocityUVW) -> outVelocityUVW/1
  sampletime/1 -> MATLAB Function/1(sampletime)
  MATLAB Function/1(outPositionLLA) -> outPositionLLA/1

== system AVE_Library/Essential/Network/Compare IP ==
  IP1 : Inport  OutDataTypeStr=uint8  PortDimensions=4
  IP2 : Inport  Port=2  OutDataTypeStr=uint8  PortDimensions=4
  Logical Operator : Logic  Inputs=4  AllPortsSameDT=off  OutDataTypeStr=boolean
  Relational Operator{,1..3} (4 alike) : RelationalOperator  Operator===  OutDataTypeStr=boolean  RndMeth=Simplest
  Selector : Selector  InputPortWidth=4  IndexOptions=Index vector (dialog)  Indices=1  OutputSizes=1
  Selector1 : Selector  InputPortWidth=4  IndexOptions=Index vector (dialog)  Indices=1  OutputSizes=1
  Selector2 : Selector  InputPortWidth=4  IndexOptions=Index vector (dialog)  Indices=2  OutputSizes=1
  Selector3 : Selector  InputPortWidth=4  IndexOptions=Index vector (dialog)  Indices=2  OutputSizes=1
  Selector4 : Selector  InputPortWidth=4  IndexOptions=Index vector (dialog)  Indices=3  OutputSizes=1
  Selector5 : Selector  InputPortWidth=4  IndexOptions=Index vector (dialog)  Indices=3  OutputSizes=1
  Selector6 : Selector  InputPortWidth=4  IndexOptions=Index vector (dialog)  Indices=4  OutputSizes=1
  Selector7 : Selector  InputPortWidth=4  IndexOptions=Index vector (dialog)  Indices=4  OutputSizes=1
  equal : Outport  VectorParamsAs1DForOutWhenUnconnected=off
  wires:
  IP2/1 -> Selector1/1, Selector7/1, Selector5/1, Selector3/1
  IP1/1 -> Selector/1, Selector2/1, Selector6/1, Selector4/1
  Selector7/1 -> Relational Operator3/2
  Selector6/1 -> Relational Operator3/1
  Selector5/1 -> Relational Operator2/2
  Selector4/1 -> Relational Operator2/1
  Selector3/1 -> Relational Operator1/2
  Selector2/1 -> Relational Operator1/1
  Selector1/1 -> Relational Operator/2
  Selector/1 -> Relational Operator/1
  Logical Operator/1 -> equal/1
  Relational Operator/1 -> Logical Operator/1
  Relational Operator1/1 -> Logical Operator/2
  Relational Operator2/1 -> Logical Operator/3
  Relational Operator3/1 -> Logical Operator/4

== system AVE_Library/Essential/Network/Message MUX ==
  bytesX : Inport  OutDataTypeStr=uint8
  lengthX : Inport  Port=2  OutDataTypeStr=uint32  PortDimensions=1
  bytesY : Inport  Port=3  OutDataTypeStr=uint8
  lengthY : Inport  Port=4  OutDataTypeStr=uint32  PortDimensions=1
  Add : Sum
  Assignment : Assignment  DiagnosticForDimensions=Warning  IndexOptions=Starting index (port)  Indices=1  OutputSizes=1
  Bias : Bias  Bias=1  SaturateOnIntegerOverflow=off
  Min : MinMax  Inputs=2
  Min1 : MinMax  Inputs=2
  Vector Concatenate : Concatenate
  Width : Width  DataType=uint32
  Width1 : Width  DataType=uint32
  bytesXY : Outport  OutDataTypeStr=uint8
  lengthXY : Outport  Port=2  OutDataTypeStr=uint32  PortDimensions=1
  wires:
  Add/1 -> lengthXY/1
  lengthX/1 -> Min/2
  Assignment/1 -> bytesXY/1
  Width/1 -> Min/1
  Vector Concatenate/1 -> Assignment/1
  Bias/1 -> Assignment/3
  bytesX/1 -> Width/1, Vector Concatenate/1
  lengthY/1 -> Min1/2
  Width1/1 -> Min1/1
  Min/1 -> Add/1, Bias/1
  bytesY/1 -> Vector Concatenate/2, Assignment/2, Width1/1
  Min1/1 -> Add/2

== system AVE_Library/Essential/Network/Swap Double Host To Network ==
  note: Check endianess of this machine
      | (only swap on little-endian-based machines)
  in : Inport  OutDataTypeStr=double
  Byte Pack1 : etargetslib/Byte Pack  datatypes={'uint16'}  byteAlign=1
  Constant : Constant  Value=uint16(1)
  Selector2 : Selector  InputPortWidth=2  IndexOptions=Index vector (dialog)  Indices=1  OutputSizes=1
  Swap Each Element : Subsystem  TreatAsAtomicUnit=on
  Switch : Switch  Criteria=u2 ~= 0  SaturateOnIntegerOverflow=off  InputSameDT=off
  out : Outport  OutDataTypeStr=double  VectorParamsAs1DForOutWhenUnconnected=off
  wires:
  Selector2/1 -> Switch/2
  Switch/1 -> out/1
  in/1 -> Switch/3, Swap Each Element/1(in)
  Byte Pack1/1 -> Selector2/1
  Constant/1 -> Byte Pack1/1
  Swap Each Element/1(out) -> Switch/1

== system AVE_Library/Essential/Network/Swap Float Host To Network ==
  note: Check endianess of this machine
      | (only swap on little-endian-based machines)
  in : Inport  OutDataTypeStr=single
  Byte Pack1 : etargetslib/Byte Pack  datatypes={'uint16'}  byteAlign=1
  Constant : Constant  Value=uint16(1)
  Selector2 : Selector  InputPortWidth=2  IndexOptions=Index vector (dialog)  Indices=1  OutputSizes=1
  Swap Each Element : Subsystem  TreatAsAtomicUnit=on
  Switch : Switch  Criteria=u2 ~= 0  SaturateOnIntegerOverflow=off  InputSameDT=off
  out : Outport  OutDataTypeStr=single
  wires:
  Swap Each Element/1(out) -> Switch/1
  Switch/1 -> out/1
  Selector2/1 -> Switch/2
  in/1 -> Switch/3, Swap Each Element/1(in)
  Byte Pack1/1 -> Selector2/1
  Constant/1 -> Byte Pack1/1

== system AVE_Library/Essential/Network/Swap Int16 Host To Network ==
  note: Check endianess of this machine
      | (only swap on little-endian-based machines)
  in : Inport  OutDataTypeStr=int16
  Byte Pack1 : etargetslib/Byte Pack  datatypes={'uint16'}  byteAlign=1
  Constant : Constant  Value=uint16(1)
  Selector2 : Selector  InputPortWidth=2  IndexOptions=Index vector (dialog)  Indices=1  OutputSizes=1
  Swap Each Element : Subsystem  TreatAsAtomicUnit=on
  Switch : Switch  Criteria=u2 ~= 0  SaturateOnIntegerOverflow=off  InputSameDT=off
  out : Outport  OutDataTypeStr=int16
  wires:
  Swap Each Element/1(out) -> Switch/1
  Switch/1 -> out/1
  Selector2/1 -> Switch/2
  in/1 -> Switch/3, Swap Each Element/1(in)
  Byte Pack1/1 -> Selector2/1
  Constant/1 -> Byte Pack1/1

== system AVE_Library/Essential/Network/Swap Int32 Host To Network ==
  note: Check endianess of this machine
      | (only swap on little-endian-based machines)
  in : Inport  OutDataTypeStr=int32
  Byte Pack1 : etargetslib/Byte Pack  datatypes={'uint16'}  byteAlign=1
  Constant : Constant  Value=uint16(1)
  Selector2 : Selector  InputPortWidth=2  IndexOptions=Index vector (dialog)  Indices=1  OutputSizes=1
  Swap Each Element : Subsystem  TreatAsAtomicUnit=on
  Switch : Switch  Criteria=u2 ~= 0  SaturateOnIntegerOverflow=off  InputSameDT=off
  out : Outport  OutDataTypeStr=int32
  wires:
  in/1 -> Switch/3, Swap Each Element/1(in)
  Switch/1 -> out/1
  Constant/1 -> Byte Pack1/1
  Byte Pack1/1 -> Selector2/1
  Selector2/1 -> Switch/2
  Swap Each Element/1(out) -> Switch/1

== system AVE_Library/Essential/Network/Swap Uint16 Host To Network ==
  note: Check endianess of this machine
      | (only swap on little-endian-based machines)
  in : Inport  OutDataTypeStr=uint16
  Byte Pack1 : etargetslib/Byte Pack  datatypes={'uint16'}  byteAlign=1
  Constant : Constant  Value=uint16(1)
  Selector2 : Selector  InputPortWidth=2  IndexOptions=Index vector (dialog)  Indices=1  OutputSizes=1
  Swap Each Element : Subsystem  TreatAsAtomicUnit=on
  Switch : Switch  Criteria=u2 ~= 0  SaturateOnIntegerOverflow=off  InputSameDT=off
  out : Outport  OutDataTypeStr=uint16
  wires:
  in/1 -> Switch/3, Swap Each Element/1(in)
  Switch/1 -> out/1
  Constant/1 -> Byte Pack1/1
  Byte Pack1/1 -> Selector2/1
  Selector2/1 -> Switch/2
  Swap Each Element/1(out) -> Switch/1

== system AVE_Library/Essential/Network/Swap Uint32 Host To Network ==
  note: Check endianess of this machine
      | (only swap on little-endian-based machines)
  in : Inport  OutDataTypeStr=uint32
  Byte Pack1 : etargetslib/Byte Pack  datatypes={'uint16'}  byteAlign=1
  Constant : Constant  Value=uint16(1)
  Selector2 : Selector  InputPortWidth=2  IndexOptions=Index vector (dialog)  Indices=1  OutputSizes=1
  Swap Each Element : Subsystem  TreatAsAtomicUnit=on
  Switch : Switch  Criteria=u2 ~= 0  SaturateOnIntegerOverflow=off  InputSameDT=off
  out : Outport  OutDataTypeStr=uint32
  wires:
  Swap Each Element/1(out) -> Switch/1
  Selector2/1 -> Switch/2
  Byte Pack1/1 -> Selector2/1
  Switch/1 -> out/1
  in/1 -> Switch/3, Swap Each Element/1(in)
  Constant/1 -> Byte Pack1/1

== system AVE_Library/Essential/Signal Logics/Hold Timeout ==
  time : Inport  OutDataTypeStr=double  Unit=s  PortDimensions=1
  timeToHold : Inport  Port=2  OutDataTypeStr=double  Unit=s  PortDimensions=1
  tfTimeout : Inport  Port=3  OutDataTypeStr=boolean  PortDimensions=1
  Abs : Abs  SaturateOnIntegerOverflow=off
  MATLAB Function : MATLAB Function  TreatAsAtomicUnit=on
  tfHoldTimeout : Outport  OutDataTypeStr=boolean  PortDimensions=1
  wires:
  timeToHold/1 -> Abs/1
  MATLAB Function/1(tfHoldTimeout) -> tfHoldTimeout/1
  Abs/1 -> MATLAB Function/3(timeHold)
  time/1 -> MATLAB Function/1(time)
  tfTimeout/1 -> MATLAB Function/2(tfTimeout)
